simulink model "aufg6"  (R2024a)
settings: Solver=FixedStepDiscrete  StartTime=0.0  StopTime=2400  FixedStep=1  RelTol=1e-3
libraries: simulink x1
settings Model: Creator=Soeren  LastModifiedBy=Soeren

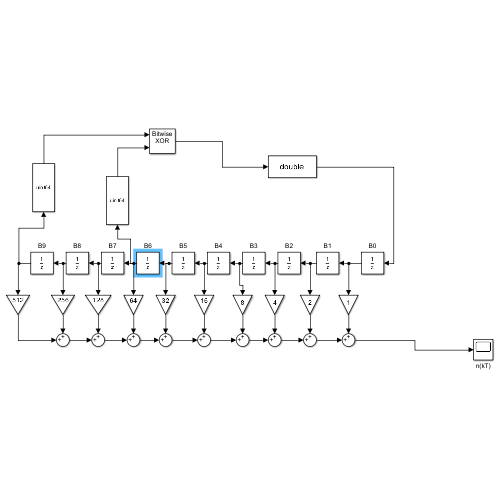
[thumbnail: Simulink's stored preview of the top-level diagram]
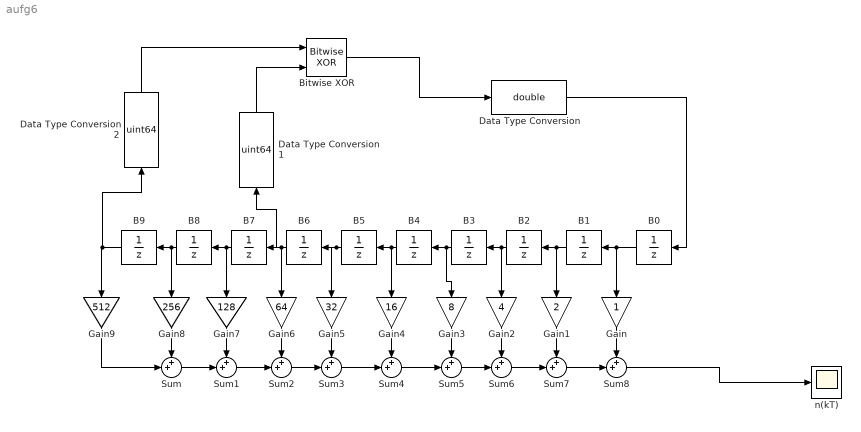
== system aufg6 ==
  B{0..9} (10 alike) : UnitDelay  InitialCondition=0000011001  HasFrameUpgradeWarning=on
  Bitwise XOR : simulink/Logic and Bit Operations/Bitwise Operator  logicop=XOR  UseBitMask=off  NumInputPorts=2  BitMask=bin2dec('11011001')  BitMaskRealWorld=Stored Integer
      settings: LibrarySourceBlock=|
      | simulink/Quick Insert/Logic and Bit
      | Operations/Bitwise XOR
  Data Type Conversion : DataTypeConversion  OutDataTypeStr=double  SaturateOnIntegerOverflow=off  RndMeth=Floor
  Data Type Conversion1 : DataTypeConversion  OutDataTypeStr=uint64  SaturateOnIntegerOverflow=off  RndMeth=Floor
  Data Type Conversion2 : DataTypeConversion  OutDataTypeStr=uint64  SaturateOnIntegerOverflow=off  RndMeth=Floor
  Gain : Gain
  Gain1 : Gain  Gain=2
  Gain2 : Gain  Gain=4
  Gain3 : Gain  Gain=8
  Gain4 : Gain  Gain=16
  Gain5 : Gain  Gain=32
  Gain6 : Gain  Gain=64
  Gain7 : Gain  Gain=128
  Gain8 : Gain  Gain=256
  Gain9 : Gain  Gain=512
  Sum{,1..8} (9 alike) : Sum  Inputs=++|
  n(kT) : Scope
  wires:
  Bitwise XOR/1 -> Data Type Conversion/1
  Gain8/1 -> Sum/1
  Gain9/1 -> Sum/2
  Gain7/1 -> Sum1/1
  Sum/1 -> Sum1/2
  Gain6/1 -> Sum2/1
  Sum1/1 -> Sum2/2
  Sum2/1 -> Sum3/2
  Gain5/1 -> Sum3/1
  Sum3/1 -> Sum4/2
  Gain4/1 -> Sum4/1
  Sum4/1 -> Sum5/2
  Gain3/1 -> Sum5/1
  Sum5/1 -> Sum6/2
  Gain2/1 -> Sum6/1
  Sum6/1 -> Sum7/2
  Gain1/1 -> Sum7/1
  Sum7/1 -> Sum8/2
  Gain/1 -> Sum8/1
  Sum8/1 -> n(kT)/1
  B0/1 -> Gain/1, B1/1
  B1/1 -> Gain1/1, B2/1
  B2/1 -> Gain2/1, B3/1
  B3/1 -> Gain3/1, B4/1
  B4/1 -> Gain4/1, B5/1
  B5/1 -> Gain5/1, B6/1
  B6/1 -> Data Type Conversion1/1, Gain6/1, B7/1
  B7/1 -> Gain7/1, B8/1
  B8/1 -> Gain8/1, B9/1
  B9/1 -> Data Type Conversion2/1, Gain9/1
  Data Type Conversion/1 -> B0/1
  Data Type Conversion1/1 -> Bitwise XOR/2
  Data Type Conversion2/1 -> Bitwise XOR/1
